simulink model "pro5"  (R2020a)
settings: Solver=VariableStepAuto  StartTime=0.0  StopTime=10.0  RelTol=1e-3
undefined symbols (not defined in the file): c, R
settings Model: Creator=aa  LastModifiedBy=aa

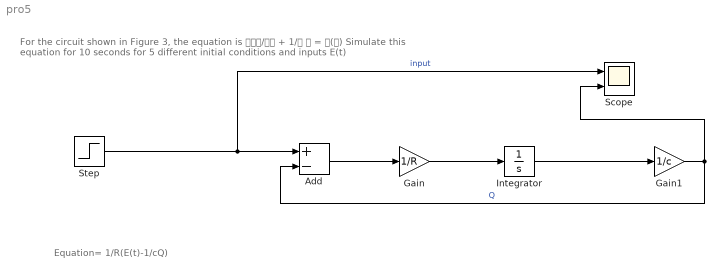
== system pro5 ==
  note: Equation= 1/R(E(t)-1/cQ)
  note: For the circuit shown in Figure 3, the equation is 𝑅𝑑𝑄/𝑑𝑡 + 1/𝐶 𝑄 = 𝐸(𝑡)
      | Simulate this equation for 10 seconds for 5 different initial conditions and inputs E(t)
  Add : Sum  Inputs=+-
  Gain : Gain  Gain=1/R
  Gain1 : Gain  Gain=1/c
  Integrator : Integrator
  Scope : Scope  NumInputPorts=2
  Step : Step  SampleTime=0
  wires:
  Step/1 -> Scope/1, Add/1  "input"
  Gain/1 -> Integrator/1
  Integrator/1 -> Gain1/1
  Gain1/1 -> Scope/2, Add/2  "Q"
  Add/1 -> Gain/1
